simulink model "HSat_orbit_merged_maria"  (R2023b)
settings: Solver=FixedStepAuto  StartTime=0  StopTime=86400*900  MaxStep=3600  RelTol=1e-3  EnableMultiTasking=on
values from neighbouring files (symbols this model uses):
  alpha_acc = sqrt(0.7)    [HSat_op_setup_merged_maria.m]    (also in init_orbit_analysis_with_drag_loss.m)
  ext_ENV_G = 6.674e-11    [HSat_op_setup.m]    (also in HSat_op_setup_merged_maria.m)
  ext_ENV_muEarth = 3.986005e14    (= 398600500000000)    [GEO_insertion_setup.m]    (also in HSat_op_setup.m; HSat_op_setup_merged_maria.m; init_orbit_analysis_with_drag_loss.m)
  ext_ENV_Re = 6.37813700*10^6    (= 6378137)    [HSat_op_setup.m]    (also in HSat_op_setup_merged_maria.m)
  ext_EOR_atmosphere_end = 1000e3    (= 1000000)    [HSat_op_setup.m]    (also in HSat_op_setup_merged_maria.m)
  ext_EOR_perigeeraise_end = 600e3    (= 600000)    [HSat_op_setup.m]    (also in HSat_op_setup_merged_maria.m)
  ext_Main_initDate_IC_T = sim_start    [HSat_op_setup.m]    (also in HSat_op_setup_merged_maria.m)
  ext_SC_activecorr_COE_ECI = [1, 1, 1, 0, 0, 0, 0, 0 ]    [HSat_op_setup.m]    (also in HSat_op_setup_merged_maria.m)
  ext_SC_balanced_COE_ECI = [ .500    0.70    1.100 1 1]    [HSat_op_setup.m]    (also in HSat_op_setup_merged_maria.m = [ 0.10 2.10 1.40    1.0000    1.0000]; launch_settings.m)
  ext_SC_cutofferror_COE_ECI = [150e3, .01, 0.1*pi/180, .1*pi/180,.1*pi/180, 0, 0, 0]    [HSat_op_setup.m]    (also in HSat_op_setup_merged_maria.m)
  ext_SC_init_COE_ECI = [a0,ecc0,i0,an0,ap0,tran0,eccan0,ma0]    [HSat_op_setup.m]    (also in HSat_op_setup_merged_maria.m)
  ext_SC_target_COE_ECI = [a1,ecc1,i1,an1,ap1,tran1,eccan1,ma1]    [HSat_op_setup.m]    (also in HSat_op_setup_merged_maria.m)
  ext_SC_target_lambda = 67*pi/180    (= 1.16937059884)    [HSat_op_setup.m]    (also in HSat_op_setup_merged_maria.m)
  flip_timer = 2*60*60    (= 7200)    [HSat_op_setup_merged_maria.m]
  P_solar = 4.56e-6    (= 4.56e-06)    [HSat_op_setup_merged_maria.m]    (also in init_orbit_analysis_with_drag_loss.m)
  sim_SC_init_CoG_EOR_dry = [-0.00448 0.00106 0.46931]    [HSat_op_setup.m]    (also in HSat_op_setup_merged_maria.m)
  sim_SC_init_CoG_propellant = [0 0 0.24758]    [HSat_op_setup.m]    (also in HSat_op_setup_merged_maria.m)
  sim_SC_init_dry_mass = sim_SC_init_wet_mass-sim_SC_init_propellant_mass    (= 727)    [HSat_op_setup.m]    (also in HSat_op_setup_merged_maria.m = 813.7)
  sim_SC_init_MoI_EOR_wet = [ ... (first row only)    [HSat_op_setup.m]    (also in HSat_op_setup_merged_maria.m; init_orbit_analysis_with_drag_loss.m)
  sim_SC_init_wet_mass = 750    [HSat_op_setup.m]    (also in HSat_op_setup_merged_maria.m)
  sim_thrust_force = [ ... (first row only)    [HSat_op_setup.m]    (also in HSat_op_setup_merged_maria.m)
  sim_thrust_massflow = [ ... (first row only)    [HSat_op_setup.m]    (also in HSat_op_setup_merged_maria.m)
  sim_thrust_vector = [ ... (first row only)    [HSat_op_setup.m]    (also in HSat_op_setup_merged_maria.m)
  sim_thruster_position = [ ... (first row only)    [HSat_op_setup.m]    (also in HSat_op_setup_merged_maria.m)
  sim_ts_save = 60    [HSat_op_setup.m]    (also in HSat_op_setup_merged_maria.m)
  sun_pointing_SA = 0    [HSat_op_setup_merged_maria.m]    (also in init_orbit_analysis_with_drag_loss.m)
  third_body_jupiter = 1    [HSat_op_setup.m]    (also in HSat_op_setup_merged_maria.m)
  third_body_moon = 1    [HSat_op_setup.m]    (also in HSat_op_setup_merged_maria.m)
  third_body_sun = 1    [HSat_op_setup.m]    (also in HSat_op_setup_merged_maria.m)
libraries: aerolibutil x59, simulink x18, matrix_library x16, Toolbox x10, sharedtransform x9, sharedutil x5, aerolibatmos2 x1, simulink_extras x1
(part 8 of 8)

== matlab function HSat_orbit_merged_maria/Subsystem1/control/EORattitude/Subsystem4/Subsystem3/Flip satellite based on worst case faior/MATLAB Function ==
  data: scMom input; worstRwMom output; thrustVect input; isFlip output; idxMaxMom output; scInertia input
function [worstRwMom, isFlip, idxMaxMom] = RW_CONTORL(scMom, thrustVect, scInertia)
d2r = pi/180;
rwa_BU = [ cos(35.26*d2r)*cos(45*d2r), -cos(35.26*d2r)*cos(45*d2r), -cos(35.26*d2r)*cos(45*d2r), cos(35.26*d2r)*cos(45*d2r);...

    -cos(35.26*d2r)*cos(45*d2r), -cos(35.26*d2r)*cos(45*d2r),  cos(35.26*d2r)*cos(45*d2r), cos(35.26*d2r)*cos(45*d2r);...

    cos(54.74*d2r),  cos(54.74*d2r),  cos(54.74*d2r), cos(54.74*d2r)];

rwa_UB = zeros(4,3,5);

for fail = 0:4

    switch fail

        case 0

            rwa_UB(:,:,fail+1) = pinv(rwa_BU);  %pseudoinverse

        case 1

            tmp = rwa_BU;

            tmp(:,fail) = [0;0;0];

            rwa_UB(:,:,fail+1) = pinv(tmp);

        case 2

            tmp = rwa_BU;

            tmp(:,fail) = [0;0;0];

            rwa_UB(:,:,fail+1) = pinv(tmp);

        case 3

            tmp = rwa_BU;

            tmp(:,fail) = [0;0;0];

            rwa_UB(:,:,fail+1) = pinv(tmp);

        case 4

            tmp = rwa_BU;

            tmp(:,fail) = [0;0;0];

            rwa_UB(:,:,fail+1) = pinv(tmp);

    end

   

end

 

% Parameters

% - rwa_UB: use above algorithm to compute it

% - flipRate: angular rate of the flip in rad/s

% - scInertia: SC inertia matrix

% Inputs:

% - scMom: angular momentum in body frame

% - thrustVect: thrust vector in body frame

% Outputs:

% - worstRwMom: highest single RW momentum for worst configuration

% - isFlip: flag to trigger the flip

% - idxMinMom: sense of the flip


flipRate = 0.1*d2r; % 0.5 deg/s

% Add rotation momentum on both sense to total angMom

tmpAngMom = [(scMom + flipRate*scInertia*thrustVect')'; (scMom - flipRate*scInertia*thrustVect')'];

% Find the flip rotation direction that results in less momentum

[~, idxMaxMom] = max(vecnorm(tmpAngMom, 2, 2));

totalAngMom = tmpAngMom(idxMaxMom, :)'; % Total angular momentum after flip

% Find RW configuration that gives the worst momentum on a wheel

worstRwMom = 0;

for rwConf = 3

    rwMom = rwa_UB(:,:,rwConf)*totalAngMom; %rotate SC ang.mom. to reaction wheel ang. mom.

    worstRwMom = max(worstRwMom, max(abs(rwMom)));

end


% The decision to do a flip is on the worst RW mom

if worstRwMom >= 22

    isFlip = true;

else

    isFlip = false;

end

end

== matlab function HSat_orbit_merged_maria/Subsystem1/Dynamics/disturbing torques/Atmospheric model/MATLAB Function1 ==
  data: julianDate input; yr output; dayOfYear output; timeUTSeconds output
function [yr, dayOfYear, timeUTSeconds] = convertJulianDate(julianDate)
    % Define constants
    secondsInDay = 86400; % Number of seconds in a day
    
    % Calculate year and day of the year
    %J0 = datetime(julianDate, 'convertfrom','juliandate');
    %yr = year(J0);
    [yr, mon, d]= splitymd(jd2ymd(julianDate));

 
    daysInMonth = [31, 28, 31, 30, 31, 30, 31, 31, 30, 31, 30, 31];
    
    % Adjust for leap year
    if mod(yr, 4) == 0 && (mod(yr, 100) ~= 0 || mod(yr, 400) == 0)
        daysInMonth(2) = 29; % February has 29 days in a leap year
    end
   
    
    dayOfYear = sum(daysInMonth(1:mon - 1)) + d;

    
    % Calculate time in UT seconds
    fractionalDay = julianDate - floor(julianDate);
    if fractionalDay < 0.5
        timeUTSeconds = (fractionalDay+0.5) * secondsInDay;
    else
        timeUTSeconds = (fractionalDay-0.5) * secondsInDay;
    end
end
